simulink model "massDAMP"  (R2021a)
settings: Solver=FixedStepAuto  StartTime=0.0  StopTime=50  FixedStep=0.01  RelTol=1e-3
undefined symbols (not defined in the file): b, k, m, x0
settings Model: Creator=Infinity  LastModifiedBy=Infinity

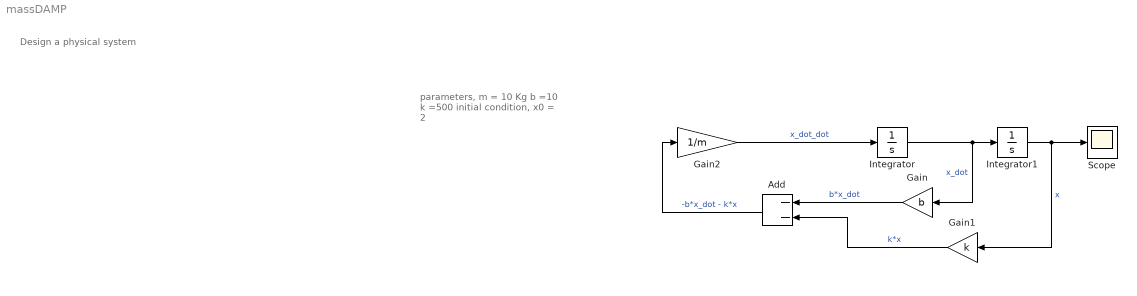
== system massDAMP ==
  note: parameters,
      |
      | m = 10 Kg
      | b =10
      | k =500
      |
      | initial condition,
      | x0 = 2
  note: Design a physical system
  Add : Sum  Inputs=--
  Gain : Gain  Gain=b
  Gain1 : Gain  Gain=k
  Gain2 : Gain  Gain=1/m
  Integrator : Integrator
  Integrator1 : Integrator  InitialCondition=x0
  Scope : Scope
  wires:
  Integrator/1 -> Gain/1, Integrator1/1  "x_dot"
  Gain2/1 -> Integrator/1  "x_dot_dot"
  Integrator1/1 -> Scope/1, Gain1/1  "x"
  Gain/1 -> Add/1  "b*x_dot"
  Gain1/1 -> Add/2  "k*x"
  Add/1 -> Gain2/1  "-b*x_dot - k*x"
